simulink model "FSK_MODEM_WITH_FFT"  (R2021b)
settings: Solver=VariableStepAuto  StartTime=0.0  StopTime=1  RelTol=1e-3
values from neighbouring files (symbols this model uses):
  fcarrier = 10000    [run_modem.m]
  fdelta = (fcarrier/100)*50    (= 5000)    [run_modem.m]
libraries: dspsrcs4 x2, commrandsrc3 x1, dspspect3 x1, dspsigops x1
settings Model: Creator=caccolillo  LastModifiedBy=caccolillo

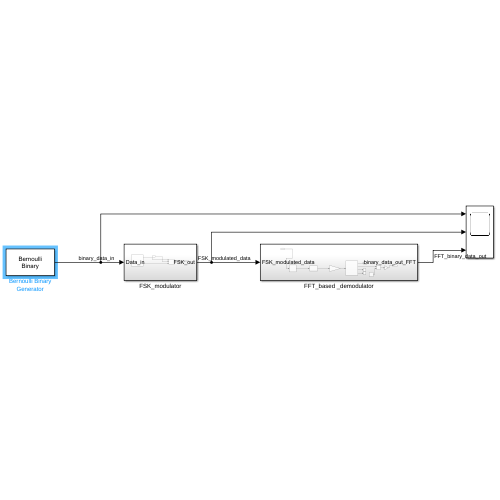
[thumbnail: Simulink's stored preview of the top-level diagram]
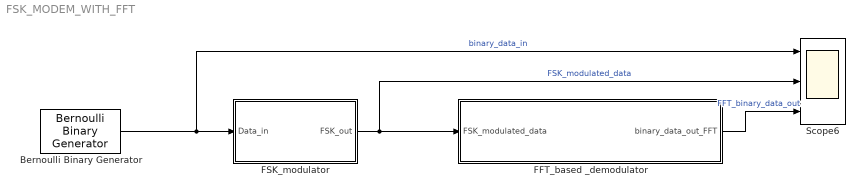
== system FSK_MODEM_WITH_FFT ==
  Bernoulli Binary Generator : commrandsrc3/Bernoulli Binary Generator  ProbabilityOfZero=0.5  SeedSource=Auto  Seed=0  SampleTime=200/fcarrier  SamplesPerFrame=1  OutputDataType=double  SimulateUsing=Interpreted execution
  FFT_based _demodulator : Subsystem
  FSK_modulator : Subsystem
  Scope6 : Scope  NumInputPorts=3
  wires:
  FSK_modulator/1(FSK_out) -> FFT_based _demodulator/1(FSK_modulated_data), Scope6/2  "FSK_modulated_data"
  Bernoulli Binary Generator/1 -> FSK_modulator/1(Data_in), Scope6/1  "binary_data_in"
  FFT_based _demodulator/1(binary_data_out_FFT) -> Scope6/3  "FFT_binary_data_out"

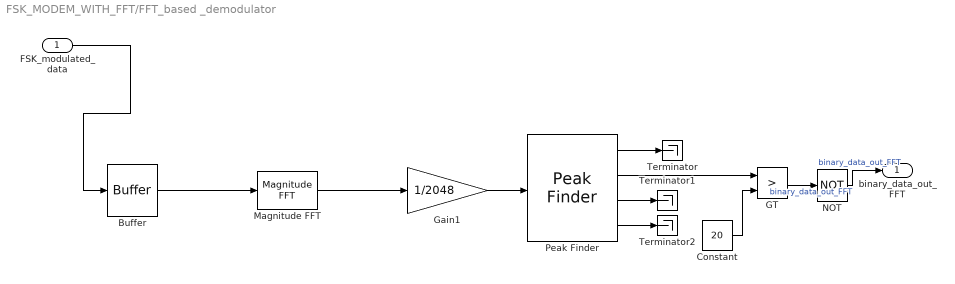
== system FSK_MODEM_WITH_FFT/FFT_based _demodulator ==
  FSK_modulated_data : Inport
  Buffer : Buffer  N=2048  OutputFrames=off
  Constant : Constant  Value=20
  GT : RelationalOperator  Operator=>  OutDataTypeStr=boolean  RndMeth=Simplest
  Gain1 : Gain  Gain=1/2048
  Magnitude FFT : dspspect3/Magnitude FFT  mag_or_magsq=Magnitude squared  FFTImplementation=Auto  fftLenInherit=off  fftsize=2048  WrapInput=on
      settings: SourceProductBaseCode=DS
  NOT : Logic  Operator=NOT  IconShape=distinctive  AllPortsSameDT=off  OutDataTypeStr=boolean
  Peak Finder : dspsigops/Peak Finder  polarity=Maxima and Minima  indexBase=Zero  outputIdx=on  outputVal=on  maxPeaks=1  NoiseDistinguish=off  thresh=0  roundingMode=Floor  overflowMode=off
      settings: SourceProductBaseCode=DS  allowOverrides=off
  Terminator : Terminator
  Terminator1 : Terminator
  Terminator2 : Terminator
  binary_data_out_FFT : Outport
  wires:
  Magnitude FFT/1 -> Gain1/1
  Peak Finder/1 -> Terminator/1
  Peak Finder/4 -> Terminator2/1
  GT/1 -> NOT/1  "binary_data_out_FFT"
  NOT/1 -> binary_data_out_FFT/1  "binary_data_out_FFT"
  Buffer/1 -> Magnitude FFT/1
  Gain1/1 -> Peak Finder/1
  Peak Finder/2 -> GT/1
  FSK_modulated_data/1 -> Buffer/1
  Constant/1 -> GT/2
  Peak Finder/3 -> Terminator1/1

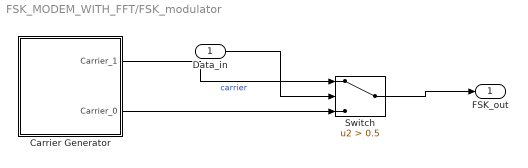
== system FSK_MODEM_WITH_FFT/FSK_modulator ==
  Data_in : Inport
  "Carrier Generator " : Subsystem
  Switch : Switch  Criteria=u2 > Threshold  Threshold=0.5
  FSK_out : Outport
  wires:
  "Carrier Generator "/1(Carrier_1) -> Switch/1  "carrier"
  "Carrier Generator "/2(Carrier_0) -> Switch/3
  Switch/1 -> FSK_out/1
  Data_in/1 -> Switch/2

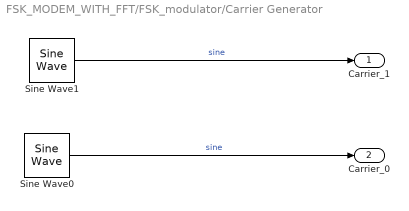
== system FSK_MODEM_WITH_FFT/FSK_modulator/Carrier Generator  ==
  Sine Wave0 : dspsrcs4/Sine Wave  Amplitude=1  Frequency=fcarrier+fdelta  Phase=0  SampleMode=Discrete  OutComplex=Real  CompMethod=Trigonometric fcn  TableSize=Speed  SampleTime=1/(100*fcarrier)  SamplesPerFrame=1  ResetState=Restart at time zero  OutputFrames=off  dataType=double  wordLen=16  udDataType=sfix(16)  fracBitsMode=Best precision  numFracBits=15  OutDataTypeStr=double  LastOutDataTypeStr=double
  Sine Wave1 : dspsrcs4/Sine Wave  Amplitude=1  Frequency=fcarrier  Phase=0  SampleMode=Discrete  OutComplex=Real  CompMethod=Trigonometric fcn  TableSize=Speed  SampleTime=1/(100*fcarrier)  SamplesPerFrame=1  ResetState=Restart at time zero  OutputFrames=off  dataType=double  wordLen=16  udDataType=sfix(16)  fracBitsMode=Best precision  numFracBits=15  OutDataTypeStr=double  LastOutDataTypeStr=double
  Carrier_1 : Outport  VectorParamsAs1DForOutWhenUnconnected=off
  Carrier_0 : Outport  Port=2  VectorParamsAs1DForOutWhenUnconnected=off
  wires:
  Sine Wave1/1 -> Carrier_1/1  "sine"
  Sine Wave0/1 -> Carrier_0/1  "sine"
